simulink model "TriggeredSubsystem"  (R2019a)
settings: Solver=VariableStepAuto  StartTime=0.0  StopTime=10.0  RelTol=1e-3
settings Model: Creator=wuyua  LastModifiedBy=wuyua

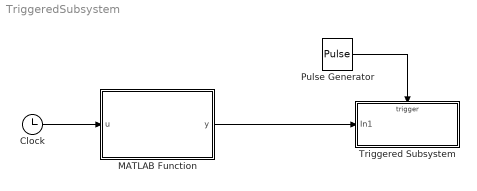
== system TriggeredSubsystem ==
  Clock : Clock
  MATLAB Function : MATLAB Function  TreatAsAtomicUnit=on
  Pulse Generator : DiscretePulseGenerator  PulseType=Time based  Period=0.2  PulseWidth=50
  Triggered Subsystem : Subsystem  TreatAsAtomicUnit=on
  wires:
  MATLAB Function/1(y) -> Triggered Subsystem/1(In1)
  Pulse Generator/1 -> Triggered Subsystem/Trigger
  Clock/1 -> MATLAB Function/1(u)

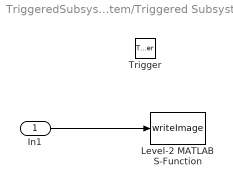
== system TriggeredSubsystem/Triggered Subsystem ==
  In1 : Inport
  Trigger : TriggerPort  VariantControl=Variant  ZeroCross=off
  Level-2 MATLAB S-Function : M-S-Function  FunctionName=writeImage
  wires:
  In1/1 -> Level-2 MATLAB S-Function/1

== matlab function TriggeredSubsystem/MATLAB Function ==
  data: u input; y output
function y = fcn(u)

y = u*ones(800,600);
